simulink model "CSMmodel"  (R2020b)
settings: Solver=VariableStepAuto  StartTime=0.0  StopTime=10.0  RelTol=1e-3
libraries: simulink_extras x3
settings Model: Creator=김예온  LastModifiedBy=김예온

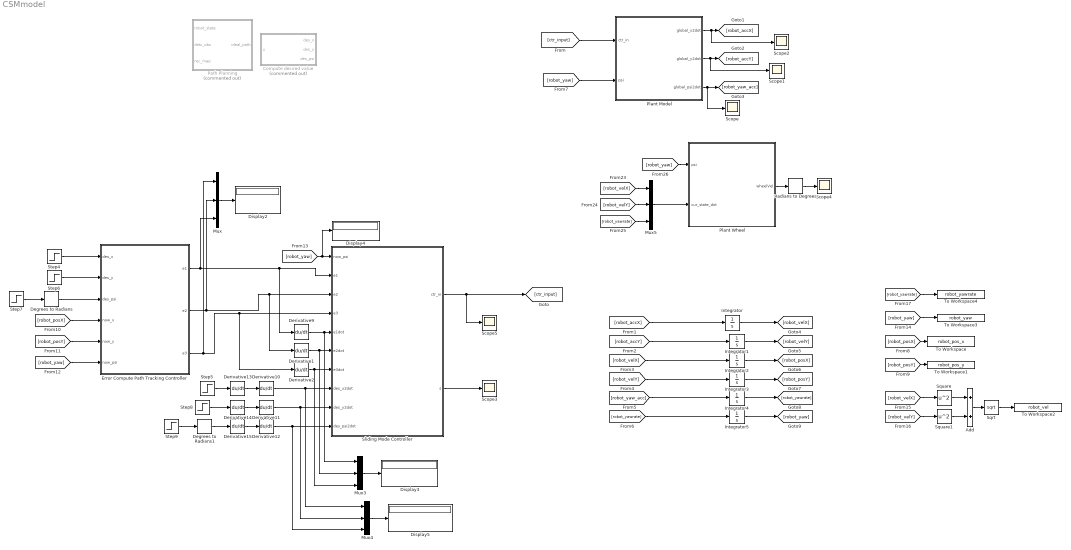
== system CSMmodel ==
  Add : Sum
  Compute desired value : MATLAB Function  Commented=on  TreatAsAtomicUnit=on
  Degrees to Radians : simulink_extras/Transformations/Degrees to Radians
  Degrees to Radians1 : simulink_extras/Transformations/Degrees to Radians
  Derivative{1..2,9..15} (9 alike) : Derivative
  Display{2..5} (4 alike) : Display
  Error Compute Path Tracking Controller : MATLAB Function  TreatAsAtomicUnit=on
  Integrator{,1..5} (6 alike) : Integrator
  Mux{,3..5} (4 alike) : Mux  Inputs=3
  Path Planning : MATLAB Function  Commented=on  TreatAsAtomicUnit=on
  Plant Model : MATLAB Function  TreatAsAtomicUnit=on
  Plant Wheel : MATLAB Function  TreatAsAtomicUnit=on
  Radians to Degrees : simulink_extras/Transformations/Radians to Degrees
  Scope{,1..5} (6 alike) : Scope
  Sliding Mode Controller : MATLAB Function  TreatAsAtomicUnit=on
  Sqrt : Sqrt  SaturateOnIntegerOverflow=on
  Square : Math  Operator=square  SaturateOnIntegerOverflow=on
  Square1 : Math  Operator=square  SaturateOnIntegerOverflow=on
  Step4 : Step  Time=0  SampleTime=0
  Step5 : Step  Time=0  SampleTime=0
  Step{6..9} (4 alike) : Step  Time=0  After=0  SampleTime=0
  To Workspace : ToWorkspace  VariableName=robot_pos_x  SaveFormat=Timeseries  SampleTime=-1
  To Workspace1 : ToWorkspace  VariableName=robot_pos_y  SaveFormat=Timeseries  SampleTime=-1
  To Workspace2 : ToWorkspace  VariableName=robot_vel  SaveFormat=Timeseries  SampleTime=-1
  To Workspace3 : ToWorkspace  VariableName=robot_yaw  SaveFormat=Timeseries  SampleTime=-1
  To Workspace4 : ToWorkspace  VariableName=robot_yawrate  SaveFormat=Timeseries  SampleTime=-1
  wires:
  Radians to Degrees/1 -> Scope4/1
  [robot_yaw] -> Plant Wheel/1(psi)
  Mux5/1 -> Plant Wheel/2(cur_state_dot)
  [robot_velX] -> Mux5/1
  [robot_yawrate] -> Mux5/3
  Derivative2/1 -> Mux3/3, Sliding Mode Controller/7(e3dot)
  Mux3/1 -> Display3/1
  Mux4/1 -> Display5/1
  Integrator1/1 -> [robot_velY]
  Plant Model/1(global_x2dot) -> Scope2/1, [robot_accX]
  Step7/1 -> Degrees to Radians/1
  Step4/1 -> Error Compute Path Tracking Controller/1(des_x)
  [robot_posX] -> To Workspace/1
  Square1/1 -> Add/2
  Degrees to Radians/1 -> Error Compute Path Tracking Controller/3(des_psi)
  Square/1 -> Add/1
  Derivative13/1 -> Derivative10/1
  [robot_yaw] -> To Workspace3/1
  Derivative9/1 -> Mux3/1, Sliding Mode Controller/5(e1dot)
  [robot_velY] -> Mux5/2
  Integrator3/1 -> [robot_posY]
  [robot_velX] -> Square/1
  Plant Wheel/1(wheelVel) -> Radians to Degrees/1
  Mux/1 -> Display2/1
  Step5/1 -> Derivative13/1
  Degrees to Radians1/1 -> Derivative15/1
  Error Compute Path Tracking Controller/1(e1) -> Mux/3, Sliding Mode Controller/2(e1), Derivative9/1
  Derivative14/1 -> Derivative11/1
  Derivative10/1 -> Mux4/1, Sliding Mode Controller/8(des_x2dot)
  Integrator4/1 -> [robot_yawrate]
  [robot_velY] -> Square1/1
  Sliding Mode Controller/2(s) -> Scope3/1
  Derivative12/1 -> Mux4/3, Sliding Mode Controller/10(des_psi2dot)
  Step6/1 -> Error Compute Path Tracking Controller/2(des_y)
  Derivative15/1 -> Derivative12/1
  Add/1 -> Sqrt/1
  [robot_yawrate] -> To Workspace4/1
  [robot_posY] -> To Workspace1/1
  Integrator5/1 -> [robot_yaw]
  [robot_yaw] -> Display4/1, Sliding Mode Controller/1(now_psi)
  [robot_yaw] -> Error Compute Path Tracking Controller/6(now_psi)
  [robot_posX] -> Error Compute Path Tracking Controller/4(now_x)
  Plant Model/2(global_y2dot) -> Scope1/1, [robot_accY]
  Plant Model/3(global_psi2dot) -> Scope/1, [robot_yaw_acc]
  Integrator2/1 -> [robot_posX]
  Error Compute Path Tracking Controller/2(e2) -> Mux/2, Sliding Mode Controller/3(e2), Derivative1/1
  Derivative1/1 -> Mux3/2, Sliding Mode Controller/6(e2dot)
  Sqrt/1 -> To Workspace2/1
  [robot_yaw] -> Plant Model/2(psi)
  [robot_posY] -> Error Compute Path Tracking Controller/5(now_y)
  Step8/1 -> Derivative14/1
  Integrator/1 -> [robot_velX]
  Step9/1 -> Degrees to Radians1/1
  Error Compute Path Tracking Controller/3(e3) -> Mux/1, Sliding Mode Controller/4(e3), Derivative2/1
  [ctr_input] -> Plant Model/1(ctr_in)
  Derivative11/1 -> Mux4/2, Sliding Mode Controller/9(des_y2dot)
  Sliding Mode Controller/1(ctr_in) -> [ctr_input], Scope5/1
  [robot_accX] -> Integrator/1
  [robot_accY] -> Integrator1/1
  [robot_velX] -> Integrator2/1
  [robot_velY] -> Integrator3/1
  [robot_yaw_acc] -> Integrator4/1
  [robot_yawrate] -> Integrator5/1

== matlab function CSMmodel/Plant Model ==
  data: ctr_in input; global_x2dot output; psi input; global_y2dot output; global_psi2dot output
function [global_x2dot, global_y2dot, global_psi2dot]= fcn(ctr_in, psi)
R = 0.05;   % wheel radius [m]
J1 = 0.095;%0.000625;  % nominal inertial of wheel [kgm^2]
H = [0 J1/2 0 J1/2;
     -J1/2 0 -J1/2 0;
     0 J1/2 0 J1/2;
     -J1/2 0 -J1/2 0];
hpsi_mat = h_psi(psi);
% global position Q = [x y psi]^T
% global state = Q2dot
% wheelspeed = [theta1dot theta2dot theta3dot theta4dot]^T
% global_state = R/(4*J1) * hpsi_mat * (H*ctr_in + J1*wheelacc);
global_state = R/(4*J1) * hpsi_mat * ctr_in;
% 
% if(isnan(global_state(1)))
%     global_state(1) = 0;
% end
% 
% if(isnan(global_state(2)))
%     global_state(2) = 0;
% end
%     
% if(isnan(global_state(3)))
%     global_state(3) = 0;
% end

global_x2dot = global_state(1);
global_y2dot = global_state(2);
global_psi2dot = global_state(3);
end

function mat = h_psi(psi)
% returns psi 3x4 matrix
psi = psi + pi/4;
root2 = sqrt(2);

% third row should be 1/(a+b) which will be 1/(2*rou)
mat = [-root2*sin(psi) root2*cos(psi) -root2*sin(psi) root2*cos(psi);
        root2*cos(psi) root2*sin(psi) root2*cos(psi) root2*sin(psi);
        10/3 -10/3 -10/3 10/3];
end

== matlab function CSMmodel/Compute desired value ==
  data: u input; des_x output; des_y output; des_psi output
function [des_x, des_y, des_psi]= fcn(u)

des_x=0;
des_y=0; 
des_psi=0;

== matlab function CSMmodel/Error Compute Path Tracking Controller ==
  data: des_x input; e1 output; des_y input; des_psi input; now_x input; now_y input; now_psi input; e2 output; e3 output
function [e1, e2, e3]= fcn(des_x, des_y, des_psi, now_x, now_y, now_psi)
e1 = -(now_x - des_x);
e2 = -(now_y - des_y);
e3 = -(now_psi - des_psi);
end

== matlab function CSMmodel/Path Planning ==
  data: robot_state input; ideal_path output; detc_obs input; rec_map input
function ideal_path = fcn(robot_state, detc_obs, rec_map)

ideal_path = robot_state;

== matlab function CSMmodel/Sliding Mode Controller ==
  data: now_psi input; ctr_in output; e1 input; e2 input; e3 input; e1dot input; e2dot input; e3dot input; des_x2dot input; des_y2dot input; des_psi2dot input; s output
function [ctr_in, s]= fcn(now_psi, e1, e2, e3, e1dot, e2dot, e3dot, des_x2dot, des_y2dot, des_psi2dot)
J1 = 0.095;%0.000625;  % nominal inertial of wheel [kgm^2]
R = 0.05;   % wheel radius [m]
lamda1 = 8;%1.5;
lamda2 = 8;%1.5;
lamda3 = 8;%1.5;
lamda = [lamda1 0 0; 0 lamda2 0; 0 0 lamda3];
d = 25; %[Nm] 
N = [8*d; 8*d; 4*d/0.3];

errdot = [e1dot; e2dot; e3dot];
Qr2dot = [des_x2dot; des_y2dot; des_psi2dot];

% sliding mode
s = [e1dot + lamda1*e1; e2dot + lamda2*e2; e3dot + lamda3*e3];
hpsi_inv_mat = hpsi_inv(now_psi);     

% final control input
ctr_in = hpsi_inv_mat*(4*J1/R*(Qr2dot+lamda*errdot) + diag(N)*sign(s));

end

function mat = hpsi_inv(psi)
psi = psi + pi/4;
sqrt2 = sqrt(2);
mat = 0.25 * [-sqrt2*sin(psi) sqrt2*cos(psi) 0.3;
                sqrt2*cos(psi) sqrt2*sin(psi) -0.3;
                -sqrt2*sin(psi) sqrt2*cos(psi) -0.3;
                sqrt2*cos(psi) sqrt2*sin(psi) 0.3];
end

== matlab function CSMmodel/Plant Wheel ==
  data: psi input; cur_state_dot input; wheelVel output
function wheelVel= fcn(psi, cur_state_dot)
R = 0.05;   % wheel radius [m]
hpsi_inv_mat = hpsi_inv(psi);

wheelVel = 4/R* hpsi_inv_mat * cur_state_dot;
end

function mat = hpsi_inv(psi)
psi = psi + pi/4;
sqrt2 = sqrt(2);
mat = 0.25 * [-sqrt2*sin(psi) sqrt2*cos(psi) 0.3;
                sqrt2*cos(psi) sqrt2*sin(psi) -0.3;
                -sqrt2*sin(psi) sqrt2*cos(psi) -0.3;
                sqrt2*cos(psi) sqrt2*sin(psi) 0.3];
end
